simulink model "a20210929KillSwitchCharging"  (R2021b)
settings: Solver=VariableStepAuto  StartTime=0.0  StopTime=inf  RelTol=1e-3
model workspace (MAT data in the model file):
  Ah_chg = [23.2 23.2]
  Ah_dsg = [46.4 46.4]
  R_chg = [0.512  0.512; 0.424  0.424; 0.352  0.352; 0.28  0.28]
  R_dsg = [0.128  0.128; 0.106  0.106; 0.088  0.088; 0.07  0.07]
  T = [298.15 323.15]
  V_chg = [186.88  186.88; 224.64  224.64; 247.68  247.68; 266.88  266.88]
  V_dsg = [93.44  93.44; 112.32  112.32; 123.84  123.84; 133.44  133.44]
  soc = [0 0.25 0.75 1]
libraries: fl_lib x42, nesl_utility x38, ee_lib x19, spsOnDelayLib x1
(part 2 of 2)

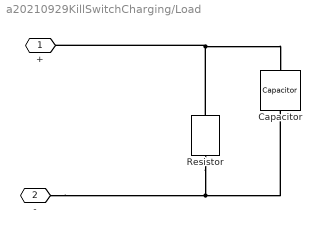
== system a20210929KillSwitchCharging/Load ==
  Capacitor : fl_lib/Electrical/Electrical Elements/Capacitor  c=6 mF  r=1e-6 Ohm  g=0 1/Ohm  i_specify=off  i_priority=None  i=0 A  i_nominal_specify=off  i_nominal_unit=A  i_nominal_value=1  v_specify=off  v_priority=None  v=0 V  v_nominal_specify=off  v_nominal_unit=V  v_nominal_value=1  vc_specify=off  vc_priority=High  vc=0 V  vc_nominal_specify=off  vc_nominal_unit=V  vc_nominal_value=1
  Resistor : ee_lib/Passive/Resistor  R=1 kOhm  R_tol=5  enable_R_tol=0  tol_distribution=1  nSigma=4  enable_operating_limits=0  operating_limit_action=2  max_working_voltage=100 V  power_rating=1 W  enable_faults=0  fault_action=1  R_faulted=inf Ohm  enable_temporal_fault=0  t_fault=1 s  enable_behavioral_fault=0  max_permissible_current=1 A  t_fail_on_current=1 s  noise_mode=0  sample_time=1e-3 s  repeatability=1  auto_seed=3499211588  user_seed=0  Tdevice=25 degC  power_derating_T1=70 degC  power_derating_T2=155 degC  operating_temperature_range_vec=[-50, 150] degC  alpha=3.93e-3 1/K  Tmeas=25 degC  thermal_mass=100 J/K  temperature_specify=off  temperature_priority=High  temperature=298.15 K  temperature_nominal_specify=off  temperature_nominal_unit=K  temperature_nominal_value=1
  + : PMIOPort  Side=Left
  - : PMIOPort  Port=2  Side=Right
  connections:
  Resistor/LConn1 -- Capacitor/LConn1 -- +/RConn1
  -/RConn1 -- Resistor/RConn1 -- Capacitor/RConn1

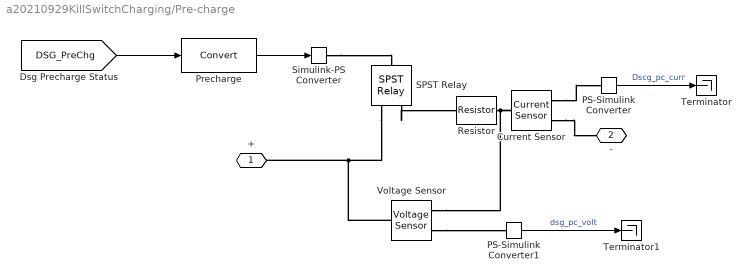
== system a20210929KillSwitchCharging/Pre-charge ==
  Current Sensor : fl_lib/Electrical/Electrical Sensors/Current Sensor
  PS-Simulink Converter : nesl_utility/PS-Simulink Converter  PhysicalDomain=network_engine_domain  SubClassName=ps_output  LeftPortType=input  RightPortType=output  PseudoPeriodic=off  Frequencies=[]  Unit=inherit  AffineConversion=off
      settings: SourceProductBaseCode=PW,SS
  PS-Simulink Converter1 : nesl_utility/PS-Simulink Converter  PhysicalDomain=network_engine_domain  SubClassName=ps_output  LeftPortType=input  RightPortType=output  PseudoPeriodic=off  Frequencies=[]  Unit=inherit  AffineConversion=off
      settings: SourceProductBaseCode=PW,SS
  Precharge : DataTypeConversion
  Resistor : ee_lib/Passive/Resistor  R=50 Ohm  R_tol=5  enable_R_tol=0  tol_distribution=1  nSigma=4  enable_operating_limits=0  operating_limit_action=2  max_working_voltage=100 V  power_rating=1 W  enable_faults=0  fault_action=1  R_faulted=inf Ohm  enable_temporal_fault=0  t_fault=1 s  enable_behavioral_fault=0  max_permissible_current=1 A  t_fail_on_current=1 s  noise_mode=0  sample_time=1e-3 s  repeatability=1  auto_seed=3360879678  user_seed=0  Tdevice=25 degC  power_derating_T1=70 degC  power_derating_T2=155 degC  operating_temperature_range_vec=[-50, 150] degC  alpha=3.93e-3 1/K  Tmeas=25 degC  thermal_mass=100 J/K  temperature_specify=off  temperature_priority=High  temperature=298.15 K  temperature_nominal_specify=off  temperature_nominal_unit=K  temperature_nominal_value=1
  SPST Relay : ee_lib/Switches & Breakers/Relays/SPST Relay  block_choices=ee.enum.controlport.ps  R_closed=0.01 Ohm  G_open=1e-8 1/Ohm  Threshold=0.5  exposemeasurement=ee.enum.exposemeasurement.hidden  V_rated=5 V  V_energize=75  V_deenergize=25  l_winding=0.08 H  r_winding=12.5 Ohm  g_winding=1e-9 1/Ohm  T_brk_C_S=0 s  T_mak_C_S=0 s  enable_faults=ee.enum.relays.enable.no  fault_action=ee.enum.relays.faultaction.none  fault_types=ee.enum.relays.faultTypes.winding  fault_condition_ps=ee.enum.relays.faultConditionSPSTps.csstuck  r_deg_closed_s=1e-9 Ohm  winding_tau_fault=1e-3 s  tau_fault=1e-3 s  enable_temporal_fault=ee.enum.relays.enable.no  t_fault_stick=1 s  t_fault_ComOpen=1 s  t_fault=1 s  enable_behavioral_fault=ee.enum.relays.enable.no  winding_max_permissible_voltage=inf V  n_fail_on_voltage=1  winding_max_permissible_current=inf A  max_permissible_current=inf A  t_fail_on_current=1 s
      settings: SourceProductBaseCode=PS  InternalSimscapePortConfiguration="{\"Bottom\":[],\"Left\":[{\"id\":\"PS\",\"label\":\"PS\",\"type\":\"input\"}],\"Right\":[{\"id\":\"S\",\"label\":\"S\",\"type\":\"foundation.electrical.electrical\"},{\"id\":\"COM\",\"label\":\"C\",\"type\":\"foundation.electrical.electrical\"}],\"Top\":[]}"
  Simulink-PS Converter : nesl_utility/Simulink-PS Converter  PhysicalDomain=network_engine_domain  SubClassName=ps_input  LeftPortType=input  RightPortType=output  PseudoPeriodic=off  Frequencies=[]  NoiseDistribution=none  NoiseParameters=[]  Unit=1  AffineConversion=off  FilteringAndDerivatives=provide  SimscapeFilterOrder=1  InputFilterTimeConstant=0.001  UdotUserProvided=0
      settings: SourceProductBaseCode=PW,SS
  Terminator : Terminator
  Terminator1 : Terminator
  Voltage Sensor : fl_lib/Electrical/Electrical Sensors/Voltage Sensor
  + : PMIOPort  Side=Left
  - : PMIOPort  Port=2  Side=Right
  wires:
  [DSG_PreChg] -> Precharge/1
  PS-Simulink Converter/1 -> Terminator/1  "Dscg_pc_curr"
  Precharge/1 -> Simulink-PS Converter/1
  PS-Simulink Converter1/1 -> Terminator1/1  "dsg_pc_volt"
  connections:
  SPST Relay/RConn1 -- Resistor/LConn1
  SPST Relay/RConn2 -- Voltage Sensor/LConn1 -- +/RConn1
  Simulink-PS Converter/RConn1 -- SPST Relay/LConn1
  Resistor/RConn1 -- Voltage Sensor/RConn2 -- Current Sensor/LConn1
  Current Sensor/RConn2 -- -/RConn1
  Current Sensor/RConn1 -- PS-Simulink Converter/LConn1
  Voltage Sensor/RConn1 -- PS-Simulink Converter1/LConn1

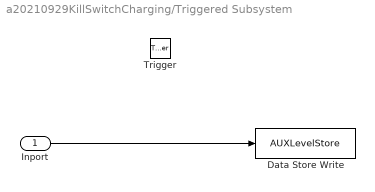
== system a20210929KillSwitchCharging/Triggered Subsystem ==
  Inport : Inport
  Trigger : TriggerPort  TriggerType=either  VariantControl=(inherit)
  Data Store Write : DataStoreWrite  DataStoreName=AUXLevelStore  IndexOptions=Index vector (dialog)  Indices=1  OutputSizes=1
  wires:
  Inport/1 -> Data Store Write/1

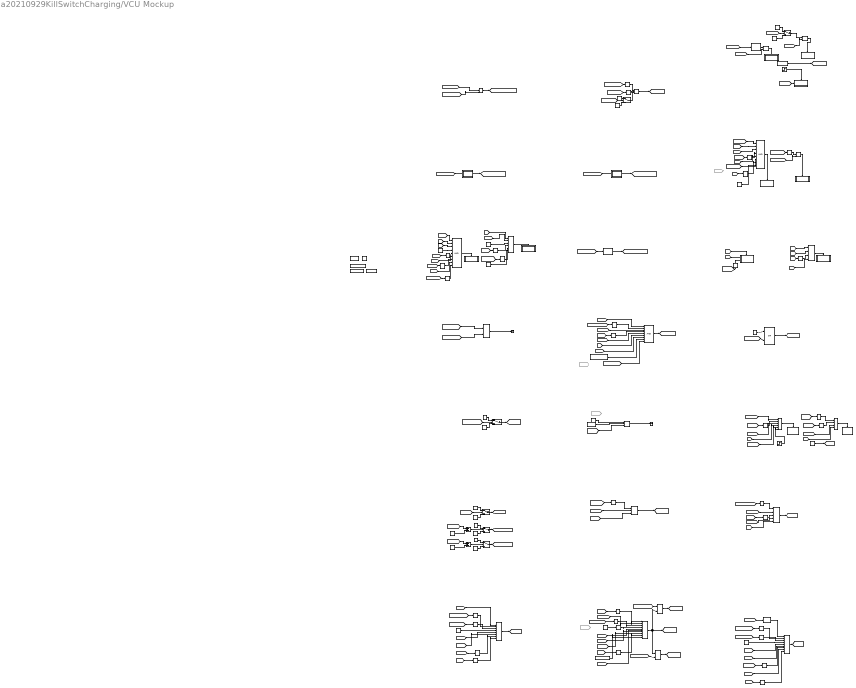
== system a20210929KillSwitchCharging/VCU Mockup ==
  note: Inputs Involved in Direct Circular Dependencies
      | Based on VCU Logic
      |
      | Charge Contactor Status
      | Discharge Contactor Status
  note: Direct Circular Dependencies
  note: Inputs Not Dependent on VCU Logic
  note: Inputs Dependent on VCU Logic
      |
      | Discharge Precharge Status
  note: Inputs Not Dependent on VCU Logic
      |
      | Key Status
      | Kill Switch Status
      | HVIL
      | Discharge Precharge
  note: Inputs Dependent on VCU Logic
      |
      | Charge Contactor Status
      | Discharge Contactor Status
      | BMS Power Passthrough From HV line to Cells
      | Charging Command
  note: Direct Circular Dependencies
      |
      | Discharge Pre Charge logic needs Charge Contator Satus to work;
      | Charge Contator logic needs Pre Charge Satuts to work
      |
      | Discharge Precharge Logic needs Discharge Contactor Status to work;
      | Discharge Contactor Logic needs Dischareg Pre Charge Status to work;
  note: EVSE Communication
  note: Charge Contactor
  note: Discharge Contactor
  note: Discharge Pre charge
  note: Charging Command
      | 0 - Discharge
      | 1 - Charge
  note: Direct Circular Dependencies
      |
      | Charge Contator logic needs Pre Charge Satuts to work;
      | Discharge Pre Charge logic needs Charge Contator Satus to work
  note: Inputs Dependent on VCU Logic
      |
      | Discharge Contactor Status
      | BMS Power Passthrough From HV line to Cells
      | Charging Command
      | Discharge Precharge
  note: Inputs Not Dependent on VCU Logic
      |
      | Key Status
      | Kill Switch Status
      | HVIL
  note: Inputs Involved in Direct Circular Dependencies
      | Based on VCU Logic
  note: Inputs Involved in Direct Circular Dependencies
      | Based on VCU Logic
      |
      | Discharge PreCharge Status
  note: Inputs Not Dependent on VCU Logic
      |
      | Charger Status
  note: Inputs Involved in Direct Circular Dependencies
      | Based on VCU Logic
  note: Inputs Dependent on VCU Logic
  note: Direct Circular Dependencies
  note: Direct Circular Dependencies
  note: Inputs Dependent on VCU Logic
      |
      | Discharge Contactor Status
      | Charging Command
      | Discharge Precharge
  note: Inputs Not Dependent on VCU Logic
      |
      | Key Status
  note: Inputs Involved in Direct Circular Dependencies
      | Based on VCU Logic
  note: BMS Power Passthrough From HV line to Cells
  note: Inputs Not Dependent on VCU Logic
      |
      | RollOver
      | HVIL
  note: Inputs Involved in Direct Circular Dependencies
      | Based on VCU Logic
  note: Inputs Dependent on VCU Logic
      |
      | AuxBatteryUp
  note: Direct Circular Dependencies
  note: Aux Battery
  note: Inputs Not Dependent on VCU Logic
      |
      | AuxBatteryChargeLevel
  note: Inputs Involved in Direct Circular Dependencies
      | Based on VCU Logic
  note: Inputs Dependent on VCU Logic
      |
      | AuxBatteryUp
  note: Direct Circular Dependencies
  note: Motor UP
  note: Inputs Not Dependent on VCU Logic
      | Kill Swicth Status
  note: Inputs Involved in Direct Circular Dependencies
      | Based on VCU Logic
  note: Inputs Dependent on VCU Logic
  note: Direct Circular Dependencies
  note: Template
  note: Inputs Not Dependent on VCU Logic
  note: Inputs Involved in Direct Circular Dependencies
      | Based on VCU Logic
  note: Inputs Dependent on VCU Logic
  note: Direct Circular Dependencies
  note: CCS Connector Solinoid
  note: Inputs Not Dependent on VCU Logic
  note: Inputs Involved in Direct Circular Dependencies
      | Based on VCU Logic
  note: Inputs Dependent on VCU Logic
  note: Direct Circular Dependencies
  note: Charging
  note: Inputs Not Dependent on VCU Logic
  note: Inputs Involved in Direct Circular Dependencies
      | Based on VCU Logic
  note: Inputs Dependent on VCU Logic
  note: Direct Circular Dependencies
  note: BMS Volt
  note: Inputs Not Dependent on VCU Logic
  note: Inputs Involved in Direct Circular Dependencies
      | Based on VCU Logic
  note: Inputs Dependent on VCU Logic
      |
      | Charge Contactor
  note: Direct Circular Dependencies
  note: VCU Memoery
  note: Ignition State
  note: Inputs Not Dependent on VCU Logic
  note: Inputs Involved in Direct Circular Dependencies
      | Based on VCU Logic
  note: Inputs Dependent on VCU Logic
  note: Direct Circular Dependencies
  note: Key Data Store
  note: Inputs Not Dependent on VCU Logic
  note: Inputs Involved in Direct Circular Dependencies
      | Based on VCU Logic
  note: Inputs Dependent on VCU Logic
  note: Direct Circular Dependencies
  note: Template
  note: Inputs Not Dependent on VCU Logic
  note: Inputs Involved in Direct Circular Dependencies
      | Based on VCU Logic
  note: Inputs Dependent on VCU Logic
  note: Direct Circular Dependencies
  note: Template
  note: Inputs Not Dependent on VCU Logic
  note: Inputs Involved in Direct Circular Dependencies
      | Based on VCU Logic
  note: Inputs Dependent on VCU Logic
  note: Direct Circular Dependencies
  note: Template
  note: Inputs Not Dependent on VCU Logic
  note: Inputs Involved in Direct Circular Dependencies
      | Based on VCU Logic
  note: Inputs Dependent on VCU Logic
  note: Direct Circular Dependencies
  note: Inputs Not Dependent on VCU Logic
  note: Inputs Involved in Direct Circular Dependencies
      | Based on VCU Logic
  note: Inputs Dependent on VCU Logic
  note: Direct Circular Dependencies
  note: Template
  note: Inputs Not Dependent on VCU Logic
  note: Inputs Involved in Direct Circular Dependencies
      | Based on VCU Logic
  note: Inputs Dependent on VCU Logic
  note: Direct Circular Dependencies
  note: AUX Battery Connected
  note: Inputs Not Dependent on VCU Logic
  note: Inputs Involved in Direct Circular Dependencies
      | Based on VCU Logic
  note: Inputs Dependent on VCU Logic
  note: Direct Circular Dependencies
  note: Screen
  note: Inputs Not Dependent on VCU Logic
  note: Inputs Involved in Direct Circular Dependencies
      | Based on VCU Logic
  note: Inputs Dependent on VCU Logic
  note: Direct Circular Dependencies
  note: AUX Battery Revival
  note: Inputs Not Dependent on VCU Logic
  note: Inputs Involved in Direct Circular Dependencies
      | Based on VCU Logic
  note: Inputs Dependent on VCU Logic
  note: Direct Circular Dependencies
  note: Enable Charging
  AND : Logic  Inputs=8  IconShape=distinctive  AllPortsSameDT=off  OutDataTypeStr=boolean
  AND1 : Logic  Inputs=6  IconShape=distinctive  AllPortsSameDT=off  OutDataTypeStr=boolean
  AND{5,10..11,16,18} (5 alike) : Logic  IconShape=distinctive  AllPortsSameDT=off  OutDataTypeStr=boolean
  AND12 : Logic  Inputs=9  IconShape=distinctive  AllPortsSameDT=off  OutDataTypeStr=boolean
  AND13 : Logic  Inputs=4  IconShape=distinctive  AllPortsSameDT=off  OutDataTypeStr=boolean
  AND14 : Logic  Inputs=4  IconShape=distinctive  AllPortsSameDT=off  OutDataTypeStr=boolean
  AND15 : Logic  Inputs=8  IconShape=distinctive  AllPortsSameDT=off  OutDataTypeStr=boolean
  AND17 : Logic  Inputs=3  IconShape=distinctive  AllPortsSameDT=off  OutDataTypeStr=boolean
  AND2 : Logic  Inputs=5  IconShape=distinctive  AllPortsSameDT=off  OutDataTypeStr=boolean
  AND3 : Logic  Inputs=10  IconShape=distinctive  AllPortsSameDT=off  OutDataTypeStr=boolean
  AND4 : Logic  Inputs=3  IconShape=distinctive  AllPortsSameDT=off  OutDataTypeStr=boolean
  AND6 : Logic  Inputs=9  IconShape=distinctive  AllPortsSameDT=off  OutDataTypeStr=boolean
  AND7 : Logic  Inputs=3  IconShape=distinctive  AllPortsSameDT=off  OutDataTypeStr=boolean
  AND8 : Logic  Inputs=9  IconShape=distinctive  AllPortsSameDT=off  OutDataTypeStr=boolean
  AND9 : Logic  Inputs=6  IconShape=distinctive  AllPortsSameDT=off  OutDataTypeStr=boolean
  Constant{,2,4..5,7,9..10,14,17..18} (10 alike) : Constant
  Constant{1,3,6,8,12..13,16} (7 alike) : Constant  Value=0
  Constant15 : Constant  Value=2
  Data Store Memory : DataStoreMemory  DataStoreName=KeyON  ReadBeforeWriteMsg=warning  WriteAfterWriteMsg=warning  WriteAfterReadMsg=warning  ShowAdditionalParam=off
  Data Store Memory1 : DataStoreMemory  DataStoreName=IgnitionState  ReadBeforeWriteMsg=warning  WriteAfterWriteMsg=warning  WriteAfterReadMsg=warning  ShowAdditionalParam=off
  Data Store Memory2 : DataStoreMemory  DataStoreName=Solinoid  ReadBeforeWriteMsg=warning  WriteAfterWriteMsg=warning  WriteAfterReadMsg=warning  ShowAdditionalParam=off
  Data Store Memory3 : DataStoreMemory  DataStoreName=EnableChargingStore  ReadBeforeWriteMsg=warning  WriteAfterWriteMsg=warning  WriteAfterReadMsg=warning  ShowAdditionalParam=off
  Data Store Memory4 : DataStoreMemory  DataStoreName=AUXRevival  ReadBeforeWriteMsg=warning  WriteAfterWriteMsg=warning  WriteAfterReadMsg=warning  InitialValue=1  ShowAdditionalParam=off
  Data Store Read : DataStoreRead  DataStoreName=IgnitionState  IndexOptions=Index vector (dialog)  Indices=1  OutputSizes=1
  Data Store Read{1,4..5,7,9} (5 alike) : DataStoreRead  DataStoreName=KeyON  IndexOptions=Index vector (dialog)  Indices=1  OutputSizes=1
  Data Store Read2 : DataStoreRead  DataStoreName=EnableChargingStore  IndexOptions=Index vector (dialog)  Indices=1  OutputSizes=1
  Data Store Read3 : DataStoreRead  DataStoreName=EnableChargingStore  IndexOptions=Index vector (dialog)  Indices=1  OutputSizes=1
  Data Store Read6 : DataStoreRead  DataStoreName=Solinoid  IndexOptions=Index vector (dialog)  Indices=1  OutputSizes=1
  Data Store Read8 : DataStoreRead  DataStoreName=AUXRevival  IndexOptions=Index vector (dialog)  Indices=1  OutputSizes=1
  From{12,26,88,100} (4 alike) : From  Commented=on  GotoTag=KillSwitch  TagVisibility=global
  MATLAB Function : MATLAB Function  TreatAsAtomicUnit=on
  MATLAB Function1 : MATLAB Function  TreatAsAtomicUnit=on
  MATLAB Function2 : MATLAB Function  TreatAsAtomicUnit=on
  MATLAB Function3 : MATLAB Function  TreatAsAtomicUnit=on
  NOT{,1..31} (32 alike) : Logic  Operator=NOT  IconShape=distinctive  AllPortsSameDT=off  OutDataTypeStr=boolean
  OR : Logic  Operator=OR  IconShape=distinctive  AllPortsSameDT=off  OutDataTypeStr=boolean
  OR1 : Logic  Operator=OR  IconShape=distinctive  AllPortsSameDT=off  OutDataTypeStr=boolean
  OR2 : Logic  Operator=OR  IconShape=distinctive  AllPortsSameDT=off  OutDataTypeStr=boolean
  On Delay : spsOnDelayLib/On Delay  DelayType=On delay  delay=2  ic=0  Ts=0
      settings: SourceProductBaseCode=PS
  Step : Step  Time=.1  SampleTime=0
  Step1 : Step  Time=.1  SampleTime=0
  Subsystem : Subsystem
  Subtract : Sum  Inputs=+-
  Subtract1 : Sum  Inputs=+-
  Switch : Switch  Criteria=u2 > Threshold
  Switch1 : Switch  Criteria=u2 > Threshold  Threshold=.10
  Switch2 : Switch  Threshold=1
  Switch3 : Switch  Criteria=u2 > Threshold  Threshold=.1
  Switch6 : Switch  Criteria=u2 ~= 0
  Switch7 : Switch  Criteria=u2 ~= 0  ZeroCross=off
  Terminator : Terminator
  Terminator1 : Terminator
  Triggered Subsystem : Subsystem  TreatAsAtomicUnit=on
  Triggered Subsystem1 : Subsystem  TreatAsAtomicUnit=on
  Triggered Subsystem2 : Subsystem  TreatAsAtomicUnit=on
  Triggered Subsystem3 : Subsystem  TreatAsAtomicUnit=on
  Triggered Subsystem4 : Subsystem  TreatAsAtomicUnit=on
  Triggered Subsystem5 : Subsystem  TreatAsAtomicUnit=on
  Triggered Subsystem6 : Subsystem  TreatAsAtomicUnit=on
  Triggered Subsystem7 : Subsystem  TreatAsAtomicUnit=on
  Triggered Subsystem8 : Subsystem  TreatAsAtomicUnit=on
  Triggered Subsystem9 : Subsystem  TreatAsAtomicUnit=on
  tag scope: AC_CHG_Cont=global, AUXRevivalON=global, BMS240Command=global, BMS=global, CHG_Cont=global, ChargeContactorON=global, ChargerConneted=global, DC_CHG_Cont=global, DSG_Cont=global, DSG_PreChg=global, DischargeContactorON=global, EvseComm=global, RunningOnAUXPower=global, ScreenON=global, SolinoidON=global
  wires:
  [ChargerMode] -> Switch/2
  Constant/1 -> Switch/1
  Constant1/1 -> Switch/3
  Switch/1 -> [ChargerConneted]
  AND/1 -> [DSG_PreChg]  "precharge"
  AND2/1 -> [EvseComm]
  [DischargeContactorON] -> NOT1/1
  NOT1/1 -> AND2/1
  [ChargerConneted] -> AND3/2
  [Key] -> NOT3/1
  Constant12/1 -> NOT5/1
  [Key] -> NOT8/1
  NOT5/1 -> AND3/4
  [BMS] -> AND3/5
  [HVIL] -> AND3/6
  [Key] -> AND/1
  [ACChargeContactorON] -> NOT7/1
  NOT7/1 -> AND/3
  NOT8/1 -> AND3/1
  Data Store Read9/1 -> AND/4  "Key ON Data Store"
  [HVIL] -> AND/6
  [RollOver] -> NOT10/1
  Constant2/1 -> Switch1/1
  [AuxBatteryChargeLevel] -> Switch1/2
  Constant3/1 -> Switch1/3
  [AuxBatteryUp] -> AND4/2
  NOT10/1 -> AND4/1
  [HVIL] -> AND4/3
  AND4/1 -> [BMS]
  Switch1/1 -> [AuxBatteryUp]
  [Key] -> NOT12/1
  NOT12/1 -> AND1/2
  [ChargerConneted] -> AND1/1
  [BMS240Command] -> AND5/1
  [EvseComm] -> AND5/2
  AND5/1 -> Terminator1/1  "Charging is Happening"
  NOT23/1 -> AND/2  "KillSwitchDischargeContactorON"
  AND7/1 -> Terminator/1  "Motor Up"
  Constant5/1 -> AND7/1
  Data Store Read/1 -> AND7/2  "Ignition State"
  AND8/1 -> Triggered Subsystem/Trigger
  [Key] -> AND9/1
  [KillSwitch] -> AND9/2
  AND9/1 -> Triggered Subsystem1/Trigger
  [Ignition] -> AND8/3
  [Key] -> AND8/2
  [KillSwitch] -> AND8/1
  Constant4/1 -> AND9/3
  [SideStand] -> NOT2/1
  NOT2/1 -> AND9/4
  [BMS] -> AND/5
  [ChargerConneted] -> NOT4/1
  NOT4/1 -> AND9/5
  [RollOver] -> NOT15/1
  AND13/1 -> Triggered Subsystem5/Trigger
  NOT15/1 -> AND13/3
  [HVIL] -> AND13/2
  [Key] -> AND13/1
  Data Store Read4/1 -> AND9/6
  Data Store Read5/1 -> AND8/4
  [DSG_PreChg] -> On Delay/1
  [SideStand] -> NOT19/1
  NOT19/1 -> AND8/5
  [HVIL] -> AND8/6
  [RollOver] -> NOT20/1
  NOT20/1 -> AND8/7
  [Key] -> Subsystem/Trigger
  [RollOver] -> NOT18/1
  [HVIL] -> Subsystem/1(Inport1)
  NOT18/1 -> Subsystem/2(Inport2)
  [BMS] -> AND8/8
  [ChargerConneted] -> NOT13/1
  NOT13/1 -> AND8/9
  [DSG_Cont] -> AND7/3
  [BMS] -> AND13/4
  [ChargerConneted] -> NOT/1
  NOT/1 -> AND/7
  [SideStand] -> AND3/7
  [RollOver] -> NOT17/1
  NOT9/1 -> AND6/7
  [ChargerConneted] -> NOT9/1
  [BMS] -> AND6/5
  [DCChargeContactorON] -> NOT22/1  "KillSwitchDischargeContactorON"
  [HVIL] -> AND6/6
  Data Store Read1/1 -> AND6/4  "Key ON Data Store"
  On Delay/1 -> AND6/1
  AND6/1 -> [DSG_Cont]
  [Key] -> AND6/8
  [ACChargeContactorON] -> NOT11/1
  NOT11/1 -> AND6/3
  MATLAB Function1/1(y) -> [DischargeContactorON]
  NOT17/1 -> AND3/8
  Data Store Read2/1 -> AND3/9
  [RollOver] -> NOT6/1
  NOT6/1 -> AND/8
  [RollOver] -> NOT21/1
  NOT21/1 -> AND6/9
  [HVIL] -> AND1/3
  [BMS] -> AND1/4
  [EvseComm] -> AND3/10
  MATLAB Function2/1(y) -> [DCChargeContactorON]
  AND11/1 -> [AC_CHG_Cont]
  AND3/1 -> AND10/1, [CHG_Cont], AND11/2  "Charge Contactor"
  AND10/1 -> [DC_CHG_Cont]
  Constant14/1 -> Switch6/3
  Constant13/1 -> Switch6/1
  [ChargerMode] -> Subtract/1
  Subtract/1 -> Switch6/2
  Constant15/1 -> Subtract/2
  Switch6/1 -> [DCChargedConnected]
  Switch7/1 -> [ACChargedConnected]
  Constant18/1 -> Subtract1/2
  Subtract1/1 -> Switch7/2
  [ChargerMode] -> Subtract1/1
  Constant16/1 -> Switch7/1
  Constant17/1 -> Switch7/3
  [ACChargedConnected] -> AND11/1
  [DCChargedConnected] -> AND10/2
  [DischargeContactorON] -> NOT24/1
  [HVIL] -> AND2/4
  [ChargerConneted] -> AND2/2
  NOT3/1 -> AND2/3
  [BMS] -> AND2/5
  [HVIL] -> AND12/5
  NOT16/1 -> AND12/4
  [ChargerConneted] -> AND12/3
  [Key] -> NOT16/1
  [DischargeContactorON] -> NOT14/1
  [BMS] -> AND12/6
  AND12/1 -> [BMS240Command]
  NOT22/1 -> AND6/2
  [DCChargeContactorON] -> NOT23/1  "KillSwitchDischargeContactorON"
  [EvseComm] -> AND12/1
  NOT14/1 -> AND12/2
  NOT24/1 -> AND3/3
  [SideStand] -> AND12/7
  Data Store Read3/1 -> AND12/8
  AND1/1 -> Triggered Subsystem2/Trigger  "Solinoid"
  [SideStand] -> AND1/5
  [BMS] -> AND14/4
  [HVIL] -> AND14/3
  [DisableCharging] -> NOT26/1
  NOT25/1 -> AND14/2
  [Key] -> NOT25/1
  NOT26/1 -> AND14/1
  AND14/1 -> Triggered Subsystem3/Trigger  "Solinoid"
  Data Store Read6/1 -> [SolinoidON]  "Solinoid"
  Step/1 -> AND1/6
  [EnableCharging] -> AND15/1
  AND15/1 -> Triggered Subsystem4/Trigger
  [RollOver] -> NOT29/1
  [SideStand] -> AND15/2
  [HVIL] -> AND15/3
  NOT29/1 -> AND15/4
  [BMS] -> AND15/5
  [ChargerConneted] -> AND15/6
  [Key] -> NOT28/1
  NOT28/1 -> AND15/7
  Constant10/1 -> AND15/8
  [ACChargeContactorON] -> OR/1
  [DCChargeContactorON] -> OR/2
  OR/1 -> [ChargeContactorON]
  AND17/1 -> [RunningOnAUXPower]
  MATLAB Function/1(y) -> [ACChargeContactorON]
  [ACChargeContactorVolatge] -> MATLAB Function/1(u)
  [DischargeContactorVolatge] -> MATLAB Function1/1(u)
  [DCChargeContactorVolatge] -> MATLAB Function2/1(u)
  Data Store Read7/1 -> OR2/1
  [ChargerConneted] -> OR2/2
  OR2/1 -> [ScreenON]
  Data Store Read8/1 -> [AUXRevivalON]
  [AUXLevel] -> MATLAB Function3/1(u)
  [AUXLevel] -> Switch2/2
  Constant6/1 -> Switch2/1
  Constant7/1 -> Switch2/3
  [ChargerConneted] -> AND16/2
  Switch2/1 -> AND16/1
  AND16/1 -> Triggered Subsystem8/Trigger
  [DischargeContactorON] -> NOT30/1
  [ChargerConneted] -> NOT31/1
  NOT31/1 -> AND17/2
  NOT30/1 -> AND17/1
  [AuxBatteryChargeLevel] -> Switch3/2
  Constant9/1 -> Switch3/1
  Constant8/1 -> Switch3/3
  Switch3/1 -> AND17/3
  MATLAB Function3/1(y) -> AND18/1
  [ChargerConneted] -> AND18/2
  AND18/1 -> Triggered Subsystem7/Trigger
  [ChargerConneted] -> Triggered Subsystem9/1(Inport)
  Step1/1 -> Triggered Subsystem9/Trigger
  [DCChargeContactorON] -> AND12/9
  [DCChargeContactorON] -> NOT27/1
  [DisableCharging] -> OR1/2
  OR1/1 -> Triggered Subsystem6/Trigger
  NOT27/1 -> OR1/1

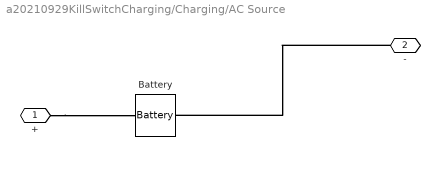
== system a20210929KillSwitchCharging/Charging/AC Source ==
  Battery : ee_lib/Sources/Battery  Vnom=240 V  prm_dir=2  R1_dis=.1 Ohm  R1_ch=1e6 Ohm  R1=.1 Ohm  prm_AH=1  AH=50 hr*A  V1=11.5 V  AH1=25 hr*A  prm_R2=1  R2=2000 Ohm  prm_dyn=1  Rp1=0.005 Ohm  tau1=30 s  Rp2=0.005 Ohm  tau2=30 s  Rp3=0.005 Ohm  tau3=30 s  Rp4=0.005 Ohm  tau4=30 s  Rp5=0.005 Ohm  tau5=30 s  prm_fade=1  N_fade=100  AH_fade=45 hr*A  R1_fade=2.02 Ohm  R1_ch_fade=2.02 Ohm  V1_fade=10.35 V  prm_age=1  prm_age_OCV=1  OCV_age=0.9  SOC_age=60  delta_time_age_vec=[0] d  temperature_age_vec=[273] K  OCV_scaling_age=2.2134e6  OCV_offset_age=1.632e6  temp_exp_age=0.515833569 V  t_exp_age=0.75  i_specify=off  i_priority=None  i=0 A  i_nominal_specify=off  i_nominal_unit=A  i_nominal_value=1  v_specify=off  v_priority=None  v=0 V  v_nominal_specify=off  v_nominal_unit=V  v_nominal_value=1  charge_specify=off  charge_priority=High  charge=50 hr*A  charge_nominal_specify=off  charge_nominal_unit=hr*A  charge_nominal_value=1  num_cycles_specify=off  num_cycles_priority=High  num_cycles=0  num_cycles_nominal_specify=off  num_cycles_nominal_unit=1  num_cycles_nominal_value=1  Tmeas=298.15 K  Tmeas_age=298.15 K  Vnom_T2=12 V  R1_T2=2.2 Ohm  R1_T2_dis=2.2 Ohm  R1_T2_ch=2.2 Ohm  V1_T2=11.4 V  R2_T2=2200 Ohm  Rp1_T2=0.005 Ohm  tau1_T2=30 s  Rp2_T2=0.005 Ohm  tau2_T2=30 s  Rp3_T2=0.005 Ohm  tau3_T2=30 s  Rp4_T2=0.005 Ohm  tau4_T2=30 s  Rp5_T2=0.005 Ohm  tau5_T2=30 s  Tmeas2=273.15 K  thermal_mass=30000 J/K  temperature_specify=off  temperature_priority=High  temperature=298.15 K  temperature_nominal_specify=off  temperature_nominal_unit=K  temperature_nominal_value=1
  + : PMIOPort  Side=Left
  - : PMIOPort  Port=2  Side=Right
  connections:
  +/RConn1 -- Battery/LConn1
  -/RConn1 -- Battery/RConn1

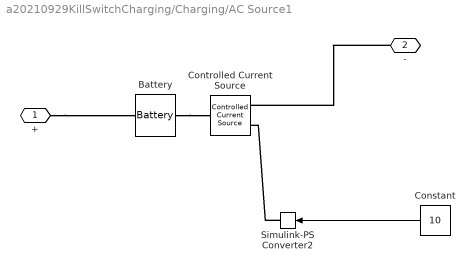
== system a20210929KillSwitchCharging/Charging/AC Source1 ==
  Battery : ee_lib/Sources/Battery  Vnom=240 V  prm_dir=1  R1_dis=2 Ohm  R1_ch=2 Ohm  R1=.1 Ohm  prm_AH=1  AH=50 hr*A  V1=11.5 V  AH1=25 hr*A  prm_R2=1  R2=2000 Ohm  prm_dyn=1  Rp1=0.005 Ohm  tau1=30 s  Rp2=0.005 Ohm  tau2=30 s  Rp3=0.005 Ohm  tau3=30 s  Rp4=0.005 Ohm  tau4=30 s  Rp5=0.005 Ohm  tau5=30 s  prm_fade=1  N_fade=100  AH_fade=45 hr*A  R1_fade=2.02 Ohm  R1_ch_fade=2.02 Ohm  V1_fade=10.35 V  prm_age=1  prm_age_OCV=1  OCV_age=0.9  SOC_age=60  delta_time_age_vec=[0] d  temperature_age_vec=[273] K  OCV_scaling_age=2.2134e6  OCV_offset_age=1.632e6  temp_exp_age=0.515833569 V  t_exp_age=0.75  i_specify=off  i_priority=None  i=0 A  i_nominal_specify=off  i_nominal_unit=A  i_nominal_value=1  v_specify=off  v_priority=None  v=0 V  v_nominal_specify=off  v_nominal_unit=V  v_nominal_value=1  charge_specify=off  charge_priority=High  charge=50 hr*A  charge_nominal_specify=off  charge_nominal_unit=hr*A  charge_nominal_value=1  num_cycles_specify=off  num_cycles_priority=High  num_cycles=0  num_cycles_nominal_specify=off  num_cycles_nominal_unit=1  num_cycles_nominal_value=1  Tmeas=298.15 K  Tmeas_age=298.15 K  Vnom_T2=12 V  R1_T2=2.2 Ohm  R1_T2_dis=2.2 Ohm  R1_T2_ch=2.2 Ohm  V1_T2=11.4 V  R2_T2=2200 Ohm  Rp1_T2=0.005 Ohm  tau1_T2=30 s  Rp2_T2=0.005 Ohm  tau2_T2=30 s  Rp3_T2=0.005 Ohm  tau3_T2=30 s  Rp4_T2=0.005 Ohm  tau4_T2=30 s  Rp5_T2=0.005 Ohm  tau5_T2=30 s  Tmeas2=273.15 K  thermal_mass=30000 J/K  temperature_specify=off  temperature_priority=High  temperature=298.15 K  temperature_nominal_specify=off  temperature_nominal_unit=K  temperature_nominal_value=1
  Constant : Constant  Value=10
  Controlled Current Source : fl_lib/Electrical/Electrical Sources/Controlled Current Source
  Simulink-PS Converter2 : nesl_utility/Simulink-PS Converter  PhysicalDomain=network_engine_domain  SubClassName=ps_input  LeftPortType=input  RightPortType=output  PseudoPeriodic=off  Frequencies=[]  NoiseDistribution=none  NoiseParameters=[]  Unit=1  AffineConversion=off  FilteringAndDerivatives=provide  SimscapeFilterOrder=1  InputFilterTimeConstant=0.001  UdotUserProvided=0
      settings: SourceProductBaseCode=PW,SS
  + : PMIOPort  Side=Left
  - : PMIOPort  Port=2  Side=Right
  wires:
  Constant/1 -> Simulink-PS Converter2/1
  connections:
  Battery/RConn1 -- Controlled Current Source/LConn1
  Simulink-PS Converter2/RConn1 -- Controlled Current Source/RConn1
  -/RConn1 -- Controlled Current Source/RConn2
  +/RConn1 -- Battery/LConn1

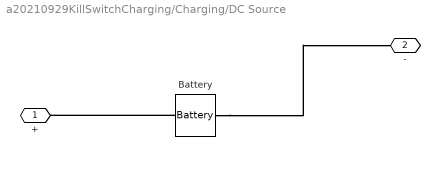
== system a20210929KillSwitchCharging/Charging/DC Source ==
  Battery : ee_lib/Sources/Battery  Vnom=240 V  prm_dir=2  R1_dis=.1 Ohm  R1_ch=1e6 Ohm  R1=.1 Ohm  prm_AH=1  AH=50 hr*A  V1=11.5 V  AH1=25 hr*A  prm_R2=1  R2=2000 Ohm  prm_dyn=1  Rp1=0.005 Ohm  tau1=30 s  Rp2=0.005 Ohm  tau2=30 s  Rp3=0.005 Ohm  tau3=30 s  Rp4=0.005 Ohm  tau4=30 s  Rp5=0.005 Ohm  tau5=30 s  prm_fade=1  N_fade=100  AH_fade=45 hr*A  R1_fade=2.02 Ohm  R1_ch_fade=2.02 Ohm  V1_fade=10.35 V  prm_age=1  prm_age_OCV=1  OCV_age=0.9  SOC_age=60  delta_time_age_vec=[0] d  temperature_age_vec=[273] K  OCV_scaling_age=2.2134e6  OCV_offset_age=1.632e6  temp_exp_age=0.515833569 V  t_exp_age=0.75  i_specify=off  i_priority=None  i=0 A  i_nominal_specify=off  i_nominal_unit=A  i_nominal_value=1  v_specify=off  v_priority=None  v=0 V  v_nominal_specify=off  v_nominal_unit=V  v_nominal_value=1  charge_specify=off  charge_priority=High  charge=50 hr*A  charge_nominal_specify=off  charge_nominal_unit=hr*A  charge_nominal_value=1  num_cycles_specify=off  num_cycles_priority=High  num_cycles=0  num_cycles_nominal_specify=off  num_cycles_nominal_unit=1  num_cycles_nominal_value=1  Tmeas=298.15 K  Tmeas_age=298.15 K  Vnom_T2=12 V  R1_T2=2.2 Ohm  R1_T2_dis=2.2 Ohm  R1_T2_ch=2.2 Ohm  V1_T2=11.4 V  R2_T2=2200 Ohm  Rp1_T2=0.005 Ohm  tau1_T2=30 s  Rp2_T2=0.005 Ohm  tau2_T2=30 s  Rp3_T2=0.005 Ohm  tau3_T2=30 s  Rp4_T2=0.005 Ohm  tau4_T2=30 s  Rp5_T2=0.005 Ohm  tau5_T2=30 s  Tmeas2=273.15 K  thermal_mass=30000 J/K  temperature_specify=off  temperature_priority=High  temperature=298.15 K  temperature_nominal_specify=off  temperature_nominal_unit=K  temperature_nominal_value=1
  + : PMIOPort  Side=Left
  - : PMIOPort  Port=2  Side=Right
  connections:
  Battery/LConn1 -- +/RConn1
  Battery/RConn1 -- -/RConn1

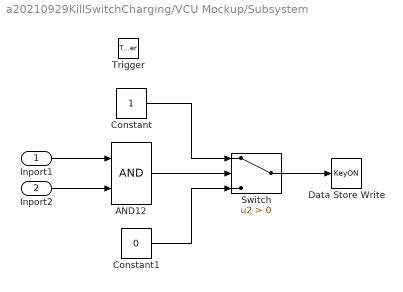
== system a20210929KillSwitchCharging/VCU Mockup/Subsystem ==
  Inport1 : Inport
  Inport2 : Inport  Port=2
  Trigger : TriggerPort  VariantControl=(inherit)  PortDimensions=1
  AND12 : Logic  IconShape=distinctive  AllPortsSameDT=off  OutDataTypeStr=boolean
  Constant : Constant
  Constant1 : Constant  Value=0
  Data Store Write : DataStoreWrite  DataStoreName=KeyON  IndexOptions=Index vector (dialog)  Indices=1  OutputSizes=1
  Switch : Switch  Criteria=u2 > Threshold
  wires:
  AND12/1 -> Switch/2
  Inport1/1 -> AND12/1
  Inport2/1 -> AND12/2
  Constant/1 -> Switch/1
  Constant1/1 -> Switch/3
  Switch/1 -> Data Store Write/1

== system a20210929KillSwitchCharging/VCU Mockup/Triggered Subsystem ==
  Trigger : TriggerPort  VariantControl=(inherit)
  Constant : Constant
  Data Store Write : DataStoreWrite  DataStoreName=IgnitionState  IndexOptions=Index vector (dialog)  Indices=1  OutputSizes=1
  wires:
  Constant/1 -> Data Store Write/1

== system a20210929KillSwitchCharging/VCU Mockup/Triggered Subsystem1 ==
  Trigger : TriggerPort  TriggerType=falling  VariantControl=(inherit)
  Constant : Constant  Value=0
  Data Store Write : DataStoreWrite  DataStoreName=IgnitionState  IndexOptions=Index vector (dialog)  Indices=1  OutputSizes=1
  wires:
  Constant/1 -> Data Store Write/1

== system a20210929KillSwitchCharging/VCU Mockup/Triggered Subsystem2 ==
  Trigger : TriggerPort  VariantControl=(inherit)
  Constant : Constant
  Data Store Write : DataStoreWrite  DataStoreName=Solinoid  IndexOptions=Index vector (dialog)  Indices=1  OutputSizes=1
  wires:
  Constant/1 -> Data Store Write/1

== system a20210929KillSwitchCharging/VCU Mockup/Triggered Subsystem3 ==
  Trigger : TriggerPort  TriggerType=falling  VariantControl=(inherit)
  Constant : Constant  Value=0
  Data Store Write : DataStoreWrite  DataStoreName=Solinoid  IndexOptions=Index vector (dialog)  Indices=1  OutputSizes=1
  wires:
  Constant/1 -> Data Store Write/1

== system a20210929KillSwitchCharging/VCU Mockup/Triggered Subsystem4 ==
  Trigger : TriggerPort  VariantControl=(inherit)
  Constant : Constant
  Data Store Write : DataStoreWrite  DataStoreName=EnableChargingStore  IndexOptions=Index vector (dialog)  Indices=1  OutputSizes=1
  wires:
  Constant/1 -> Data Store Write/1

== system a20210929KillSwitchCharging/VCU Mockup/Triggered Subsystem5 ==
  Trigger : TriggerPort  TriggerType=falling  VariantControl=(inherit)
  Constant : Constant  Value=0
  Data Store Write : DataStoreWrite  DataStoreName=KeyON  IndexOptions=Index vector (dialog)  Indices=1  OutputSizes=1
  wires:
  Constant/1 -> Data Store Write/1

== system a20210929KillSwitchCharging/VCU Mockup/Triggered Subsystem6 ==
  Trigger : TriggerPort  VariantControl=(inherit)
  Constant : Constant  Value=0
  Data Store Write : DataStoreWrite  DataStoreName=EnableChargingStore  IndexOptions=Index vector (dialog)  Indices=1  OutputSizes=1
  wires:
  Constant/1 -> Data Store Write/1

== system a20210929KillSwitchCharging/VCU Mockup/Triggered Subsystem7 ==
  Trigger : TriggerPort  VariantControl=(inherit)
  Constant : Constant
  Data Store Write : DataStoreWrite  DataStoreName=AUXRevival  IndexOptions=Index vector (dialog)  Indices=1  OutputSizes=1
  wires:
  Constant/1 -> Data Store Write/1

== system a20210929KillSwitchCharging/VCU Mockup/Triggered Subsystem8 ==
  Trigger : TriggerPort  TriggerType=falling  VariantControl=(inherit)
  Constant : Constant  Value=0
  Data Store Write : DataStoreWrite  DataStoreName=AUXRevival  IndexOptions=Index vector (dialog)  Indices=1  OutputSizes=1
  wires:
  Constant/1 -> Data Store Write/1

== system a20210929KillSwitchCharging/VCU Mockup/Triggered Subsystem9 ==
  Inport : Inport
  Trigger : TriggerPort  VariantControl=(inherit)
  Data Store Write : DataStoreWrite  DataStoreName=AUXRevival  IndexOptions=Index vector (dialog)  Indices=1  OutputSizes=1
  wires:
  Inport/1 -> Data Store Write/1

== matlab function a20210929KillSwitchCharging/VCU Mockup/MATLAB Function1 ==
  data: u input; y output
function y = fcn(u)
u=abs(u);
if u<=1
    y=1;
else
    y=0;
end

== matlab function a20210929KillSwitchCharging/VCU Mockup/MATLAB Function ==
  data: u input; y output
function y = fcn(u)
u=abs(u);
if u<=1
    y=1;
else
    y=0;
end

== matlab function a20210929KillSwitchCharging/VCU Mockup/MATLAB Function2 ==
  data: u input; y output
function y = fcn(u)
u=abs(u);
if u<=1
    y=1;
else
    y=0;
end

== matlab function a20210929KillSwitchCharging/MATLAB Function ==
  data: u input; y output
function y  = fcn(u)
if u<.10
       y=0;
elseif u>=1
       y=0;
else
    y=1;
end

== matlab function a20210929KillSwitchCharging/VCU Mockup/MATLAB Function3 ==
  data: u input; y output
function y  = fcn(u)
if u<.90
      y=1;
else
    y=0;
end

== matlab function a20210929KillSwitchCharging/Charging/MATLAB Function ==
  data: u input; y output
function y = fcn(u)
 if u==1
     y=1;
 else
     y=0;
 end

== matlab function a20210929KillSwitchCharging/Charging/MATLAB Function1 ==
  data: u input; y output
function y = fcn(u)
 if u==2
     y=1;
 else
     y=0;
 end
